simulink model "CreateOffsetSquareSignal"  (R2016b)
settings: Solver=FixedStepDiscrete  StartTime=0.0  StopTime=10.0  FixedStep=0.001  RelTol=1e-3
undefined symbols (not defined in the file): sigbuilder_block
settings Model: Creator=oelkawok  LastModifiedBy=oelkawok

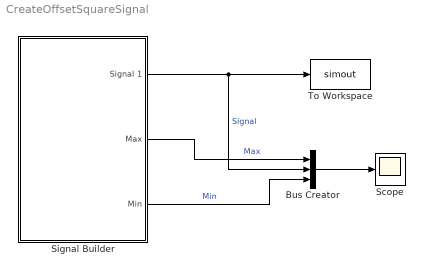
== system CreateOffsetSquareSignal ==
  Bus Creator : BusCreator  Inputs=3
  Scope : Scope
  Signal Builder : Subsystem  Tag=STV Subsys  LoadFcn=sigbuilder_block('load',[1.8 89.4 550.8 400.2 ]);  StartFcn=sigbuilder_block('start');  StopFcn=sigbuilder_block('stop');  ClipboardFcn=sigbuilder_block('clipboard');  mask(Sigbuilder block){tuvar=[0:10]}
      mask help: Simulink:masks:SigbuilderBlock_MD
      mask init:
      | if ~strcmp(get_param(bdroot(gcbh),'SimulationStatus'),'stopped') tuvar = sigbuilder_block('maskInit'); end
      settings: CopyFcn=sigbuilder_block('copy');  DeleteFcn=sigbuilder_block('delete');  ModelCloseFcn=sigbuilder_block('modelClose');  PreSaveFcn=sigbuilder_block('preSave');  PauseFcn=sigbuilder_block('pause');  ContinueFcn=sigbuilder_block('continue');  NameChangeFcn=sigbuilder_block('namechange');  OpenFcn=sigbuilder_block('open',[1.8 89.4 550.8 400.2 ]);  CloseFcn=sigbuilder_block('close');
      mask Display: plot(0, 0, 100, 100,[2, 2, 32, 32, 2], [68, 8, 8, 68, 68],[32, 2], [38, 38], [32, 19, 2],[53, 60, 44], [32, 17, 17, 2],[16, 16, 31, 31]);txt = getActiveGroup(gcbh);text(2, 100, txt,'verticalAlignment', 'top');
  To Workspace : ToWorkspace  VariableName=simout  SaveFormat=Timeseries  SampleTime=-1
  wires:
  Signal Builder/1(Signal 1) -> Bus Creator/2, To Workspace/1  "Signal"
  Bus Creator/1 -> Scope/1
  Signal Builder/2(Max) -> Bus Creator/1  "Max"
  Signal Builder/3(Min) -> Bus Creator/3  "Min"

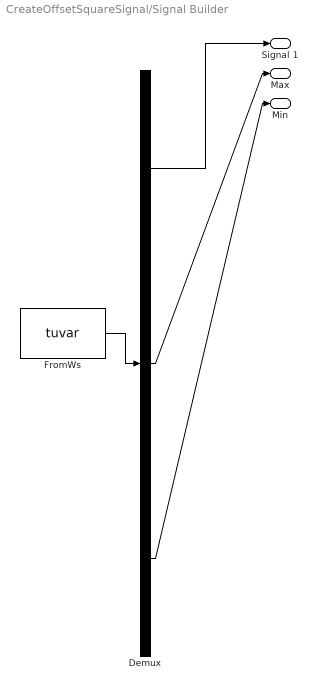
== system CreateOffsetSquareSignal/Signal Builder ==
  Demux : Demux  Tag=STV Demux  Outputs=3
  FromWs : FromWorkspace  Tag=STV FromWs  VariableName=tuvar  SampleTime=0
      SigBuilderData=|
      | common.afterFinalStr = 'Extrapolate'
      | common.sampleTime = 0
      | dataSet.timeRange = [0 10]
      | dataSet.name = 'Group 1'
      | sbobj.Groups.Name = 'Group 1'
      | sbobj.Groups.Signals(1).Name = 'Signal 1'
      | sbobj.Groups.Signals(1).XData = [0 0.88 0.88 2.2 2.2 2.88 2.88 4.4 4.4 6.68 6.68 7.22 7.22 7.64 7.64 8.82 8.82 10]
      | sbobj.Groups.Signals(1).YData = [0.58 0.58 0 0 0.64 0.64 0 0 0.88 0.88 0 0 1 1 0 0 0.52 0.52]
      | sbobj.Groups.Signals(2).Name = 'Max'
      | sbobj.Groups.Signals(2).XData = [0 0.001 0.002 0.003 0.004 0.005 0.006 0.007 0.008 0.009 0.01 0.011 ... (10001 elements, 1x10001)]
      | sbobj.Groups.Signals(2).YData = [1.08 1.08 1.08 1.08 1.08 1.08 1.08 1.08 1.08 1.08 1.08 1.08 ... (10001 elements, 1x10001)]
      | sbobj.Groups.Signals(3).Name = 'Min'
      | sbobj.Groups.Signals(3).XData = [0 0.001 0.002 0.003 0.004 0.005 0.006 0.007 0.008 0.009 0.01 0.011 ... (10001 elements, 1x10001)]
      | sbobj.Groups.Signals(3).YData = [0.08 0.08 0.08 0.08 0.08 0.08 0.08 0.08 0.08 0.08 0.08 0.08 ... (10001 elements, 1x10001)]
  Signal 1 : Outport  Tag=STV Outport
  Max : Outport  Tag=STV Outport  Port=2
  Min : Outport  Tag=STV Outport  Port=3
  wires:
  Demux/1 -> Signal 1/1
  FromWs/1 -> Demux/1
  Demux/2 -> Max/1
  Demux/3 -> Min/1
